simulink model "model1_controller_observer"  (R2022b)
settings: Solver=VariableStepAuto  StartTime=0.0  StopTime=10.0  RelTol=1e-3
InitFcn:
  | model1_init_params_stable
values from neighbouring files (symbols this model uses):
  a = 0.347    [model1_init_params_stable.m]    (also in model1_init_params_unstable.m)
  A = [ ... (first row only)    [model1_init_params_stable.m]    (also in model1_init_params_unstable.m; model2_init_params_stable.m; model2_init_params_unstable.m; model2_init_params_unstable__lqr_controller.m)
  A_obs = A-L*C    [model1_init_params_stable.m]    (also in model1_init_params_unstable.m; model2_init_params_unstable__lqr_controller.m = A_ccf-L*C_ccf)
  b = 1.02    [model1_init_params_stable.m]    (also in model1_init_params_unstable.m)
  B = [ ... (first row only)    [model1_init_params_stable.m]    (also in model1_init_params_unstable.m; model2_init_params_stable.m; model2_init_params_unstable.m; model2_init_params_unstable__lqr_controller.m)
  B_obs = [B L]    [model1_init_params_stable.m]    (also in model1_init_params_unstable.m; model2_init_params_unstable__lqr_controller.m = [B_ccf L])
  c = 0.08    [model1_init_params_stable.m]    (also in model1_init_params_unstable.m)
  C = [(V^2*h-a*c*g)*sin(lambda)/(b*h^2)*k1 a*V*sin(lambda)/(b*h)*k1]    [model1_init_params_stable.m]    (also in model1_init_params_unstable.m; model2_init_params_stable.m = [1 0 0 0]; model2_init_params_unstable.m = [1 0 0 0]; model2_init_params_unstable__lqr_controller.m = [1 0 0 0])
  C_obs = eye(length(A_obs))    [model1_init_params_stable.m]    (also in model1_init_params_unstable.m; model2_init_params_unstable__lqr_controller.m)
  D = 0    [model1_init_params_stable.m]    (also in model1_init_params_unstable.m; model2_init_params_stable.m; model2_init_params_unstable.m; model2_init_params_unstable__lqr_controller.m)
  D_obs = zeros(size(B_obs))    [model1_init_params_stable.m]    (also in model1_init_params_unstable.m; model2_init_params_unstable__lqr_controller.m)
  g = 9.81    [model1_init_params_stable.m]    (also in model1_init_params_unstable.m)
  h = 0.8603    [model1_init_params_stable.m]    (also in model1_init_params_unstable.m)
  k1 = b^2/((V^2*sin(lambda) - b*g*cos(lambda))*m*a*c*sin(lambda))    [model1_init_params_stable.m]    (also in model1_init_params_unstable.m)
  k2 = b*g/(V^2*sin(lambda) - b*g*cos(lambda))    [model1_init_params_stable.m]    (also in model1_init_params_unstable.m)
  lambda = pi/10    (= 0.314159265359)    [model1_init_params_stable.m]    (also in model1_init_params_unstable.m)
  V = 5.7    [model1_init_params_stable.m]    (also in model1_init_params_unstable.m = 3; model2_init_params_stable.m = 6.1; model2_init_params_unstable.m = 5; model2_init_params_unstable__lqr_controller.m = 5)
settings Model: Creator=neotod  LastModifiedBy=neotod

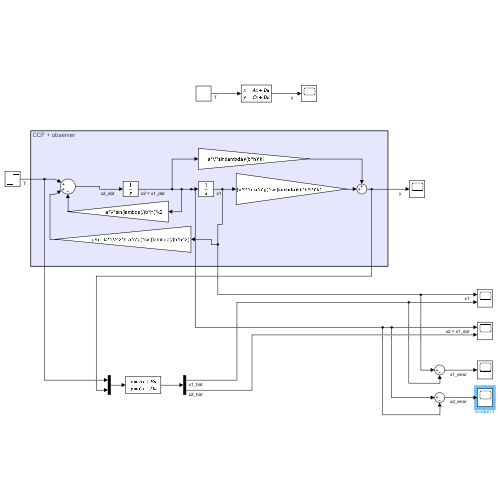
[thumbnail: Simulink's stored preview of the top-level diagram]
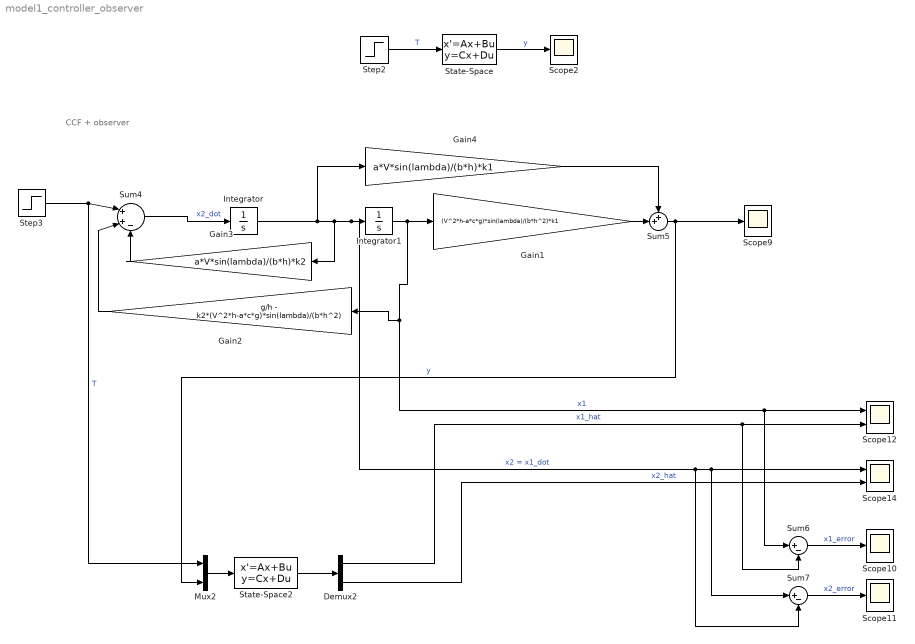
== system model1_controller_observer ==
  note: CCF + observer
  Demux2 : Demux  Outputs=2
  Gain1 : Gain  Gain=(V^2*h-a*c*g)*sin(lambda)/(b*h^2)*k1
  Gain2 : Gain  Gain=g/h - k2*(V^2*h-a*c*g)*sin(lambda)/(b*h^2)
  Gain3 : Gain  Gain=a*V*sin(lambda)/(b*h)*k2
  Gain4 : Gain  Gain=a*V*sin(lambda)/(b*h)*k1
  Integrator : Integrator
  Integrator1 : Integrator
  Mux2 : Mux  Inputs=2
  Scope{2,9..11} (4 alike) : Scope
  Scope12 : Scope  NumInputPorts=2
  Scope14 : Scope  NumInputPorts=2
  State-Space : StateSpace  A=A  B=B  C=C  D=D  InitialCondition=0
  State-Space2 : StateSpace  A=A_obs  B=B_obs  C=C_obs  D=D_obs  InitialCondition=0
  Step2 : Step  SampleTime=0
  Step3 : Step  SampleTime=0
  Sum4 : Sum  Inputs=|++-
  Sum5 : Sum  Inputs=++|
  Sum6 : Sum  Inputs=|+-
  Sum7 : Sum  Inputs=|+-
  wires:
  State-Space/1 -> Scope2/1  "y"
  Step2/1 -> State-Space/1  "T"
  Sum7/1 -> Scope11/1  "x2_error"
  Sum6/1 -> Scope10/1  "x1_error"
  Demux2/2 -> Scope14/2  "x2_hat"
  Demux2/1 -> Sum6/2, Scope12/2  "x1_hat"
  State-Space2/1 -> Demux2/1
  Mux2/1 -> State-Space2/1
  Gain1/1 -> Sum5/2
  Integrator/1 -> Gain4/1, Gain3/1, Sum7/2, Sum7/1, Scope14/1, Integrator1/1  "x2 = x1_dot"
  Gain3/1 -> Sum4/3
  Gain2/1 -> Sum4/2
  Sum5/1 -> Mux2/2, Scope9/1  "y"
  Step3/1 -> Mux2/1, Sum4/1  "T"
  Sum4/1 -> Integrator/1  "x2_dot"
  Gain4/1 -> Sum5/1
  Integrator1/1 -> Gain1/1, Sum6/1, Scope12/1, Gain2/1  "x1"
